simulink model "exp0303_sist_faltafaseterra"  (R2021b)
settings: Solver=ode23t  StartTime=0.0  StopTime=0.1  RelTol=1e-5  EnableMultiTasking=on
libraries: powerlib_extras x7, spsCurrentMeasurementLib x4, spsGroundLib x4, spsVoltageMeasurementLib x3, spsThreePhaseSeriesRLCBranchLib x2, spsThreePhaseSourceLib x1, spspowerguiLib x1
settings Model: Creator=alunos  LastModifiedBy=luang
settings SolverCC: AlgebraicLoopSolver=TrustRegion
settings DataIOCC: LimitDataPoints=on  SaveFormat=Array  SignalLoggingSaveFormat=ModelDataLogs  ReturnWorkspaceOutputs=off
settings OptimizationCC: ExpressionDepthLimit=2147483647  LifeSpan=inf
settings DebuggingCC: UnderspecifiedInitializationDetection=Classic  MergeDetectMultiDrivingBlocksExec=none  SolverPrmCheckMsg=warning  FcnCallInpInsideContextMsg=warning  StateNameClashWarn=warning  SFUnexpectedBacktrackingDiag=warning  SFNoUnconditionalDefaultTransitionDiag=warning  SFExecutionAtInitializationDiag=none  SFMachineParentedDataDiag=warning  ArithmeticOperatorsInVariantConditions=warning
settings HardwareCC: ProdBitPerPointer=32  ProdBitPerSizeT=32  ProdBitPerPtrDiffT=32  ProdLargestAtomicFloat=None  ProdIntDivRoundTo=Undefined  ProdEndianess=Unspecified  ProdWordSize=32  ProdHWDeviceType=32-bit Generic
settings ModelReferenceCC: PropagateSignalLabelsOutOfModel=off
settings SFSimCC: SimUseLocalCustomCode=off  CustomCodeUndefinedFunction=UseInterfaceOnly
settings RTWCC: RTWUseLocalCustomCode=off
settings CodeAppCC: StateflowObjectComments=on
settings GRTTargetCC: TargetLangStandard=C89/C90 (ANSI)  CombineOutputUpdateFcns=off  GRTInterface=on
settings ConfigComp: CovMetricSettings=dw  CovSaveCumulativeToWorkspaceVar=on  CovSaveSingleToWorkspaceVar=on  CovExternalEMLEnable=off

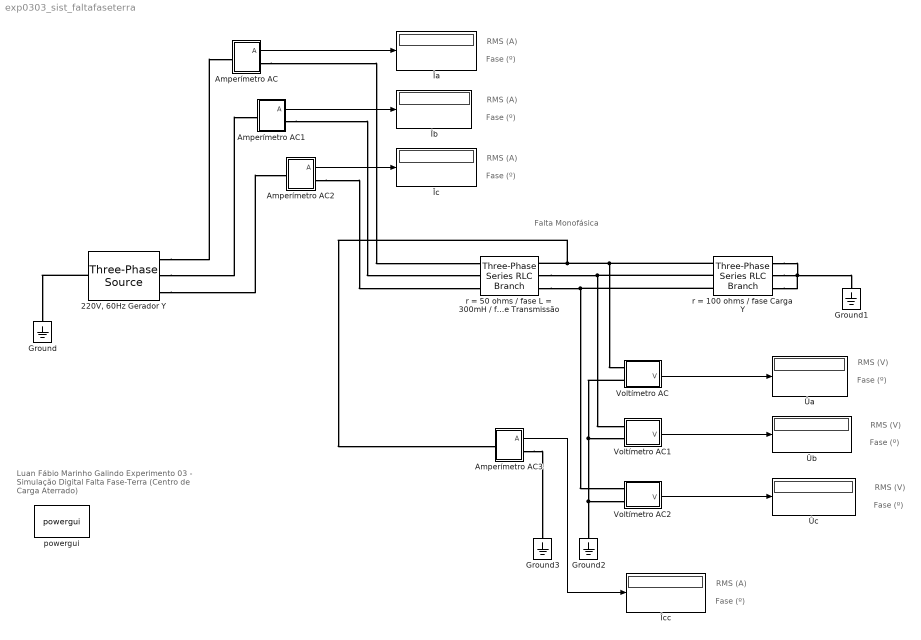
== system exp0303_sist_faltafaseterra ==
  note: Falta Monofásica
  note: RMS (A)
  note: Fase (º)
  note: RMS (A)
  note: Fase (º)
  note: RMS (A)
  note: Fase (º)
  note: RMS (V)
  note: Fase (º)
  note: RMS (V)
  note: Fase (º)
  note: RMS (V)
  note: Fase (º)
  note: Luan Fábio Marinho Galindo
      | Experimento 03 - Simulação Digital
      | Falta Fase-Terra (Centro de Carga Aterrado)
  note: RMS (A)
  note: Fase (º)
  "220V, 60Hz Gerador Y" : spsThreePhaseSourceLib/Three-Phase Source  InternalConnection=Yn  VoltagePhases=off  Voltage=220  PhaseAngle=90  Voltage_phases=[25e3 25e3 25e3]/sqrt(3)  PhaseAngles_phases=[0 -120 +120]  Frequency=60  NonIdealSource=on  SpecifyImpedance=off  Resistance=0.001  Inductance=0  ShortCircuitLevel=100e6  BaseVoltage=25e3  XRratio=7  BusType=swing  Pref=0  Qref=0  Prefabc=[10e3, 10e3, 10e3]  Qrefabc=[0, 0, 0]  Qmin=-inf  Qmax=inf
  Amperímetro AC : Subsystem
  Amperímetro AC1 : Subsystem
  Amperímetro AC2 : Subsystem
  Amperímetro AC3 : Subsystem
  Ground{,1..3} (4 alike) : spsGroundLib/Ground  LConnTagsString=a
  Voltímetro AC : Subsystem
  Voltímetro AC1 : Subsystem
  Voltímetro AC2 : Subsystem
  powergui : spspowerguiLib/powergui  Priority=1  SimulationMode=Continuous  SampleTime=50e-6  frequency=60  Iterations=50  frequencyindice=60  Pbase=100e6  ErrMax=1e-4  UnitsV=kV  UnitsW=MW  buscounter=0  FunctionMessages=off  echomessages=off  EnableUseOfTLC=off  CurrentSourceSwitches=on  DisableSnubberDevices=off  DisableRonSwitches=off  DisableVfSwitches=off  DisplayEquations=off  AutomaticDiscreteSolvers=off  SolverType=Tustin/Backward Euler (TBE)  Interpol=off  ExternalGateDelay=off  methode=off  Ts=100  x0status=blocks  SPID=off  SwTol=0  HookPort=off  NonlinearTolerance=1e-4  nMaxIteration=100  ContinueOnMaxIteration=off  RestoreLinks=warning  ResistiveCurrentMeasurement=off  Frange=[0:2:500]  Ylog=off  Xlog=on  ShowGrid=off  save=off  variable=ZData  structure=0  ZoomFFT=off  StartTime=0.0  cycles=1  DisplayStyle=1  fundamental=60  FreqAxis=off  MaxFrequency=1000  frequencyindicesteady=1  RmsSteady=1  display=off
  r = 100 ohms / fase Carga Y : spsThreePhaseSeriesRLCBranchLib/Three-Phase Series RLC Branch  LConnTagsString=A|B|C  RConnTagsString=A|B|C  BranchType=R  Resistance=100  Inductance=1e-3  Capacitance=1e-6  Measurements=None
  r = 50 ohms / fase L = 300mH / fase Linha de Transmissão : spsThreePhaseSeriesRLCBranchLib/Three-Phase Series RLC Branch  LConnTagsString=A|B|C  RConnTagsString=A|B|C  BranchType=RL  Resistance=50  Inductance=300e-3  Capacitance=1e-6  Measurements=None
  Îa : Display
      settings: Format=bank
  Îb : Display
      settings: Format=bank
  Îc : Display
      settings: Format=bank
  Îcc : Display
      settings: Format=bank
  Ûa : Display
      settings: Format=bank
  Ûb : Display
      settings: Format=bank
  Ûc : Display
      settings: Format=bank
  wires:
  Amperímetro AC/1(A) -> Îa/1
  Amperímetro AC1/1(A) -> Îb/1
  Amperímetro AC2/1(A) -> Îc/1
  Voltímetro AC/1(V) -> Ûa/1
  Voltímetro AC1/1(V) -> Ûb/1
  Voltímetro AC2/1(V) -> Ûc/1
  Amperímetro AC3/1(A) -> Îcc/1
  connections:
  "220V, 60Hz Gerador Y"/RConn1 -- Amperímetro AC/LConn1
  "220V, 60Hz Gerador Y"/RConn2 -- Amperímetro AC1/LConn1
  "220V, 60Hz Gerador Y"/RConn3 -- Amperímetro AC2/LConn1
  Amperímetro AC/RConn1 -- r = 50 ohms / fase L = 300mH / fase Linha de Transmissão/LConn1
  Amperímetro AC1/RConn1 -- r = 50 ohms / fase L = 300mH / fase Linha de Transmissão/LConn2
  Amperímetro AC2/RConn1 -- r = 50 ohms / fase L = 300mH / fase Linha de Transmissão/LConn3
  r = 100 ohms / fase Carga Y/RConn2 -- r = 100 ohms / fase Carga Y/RConn3 -- r = 100 ohms / fase Carga Y/RConn1 -- Ground1/LConn1
  Voltímetro AC/LConn1 -- r = 100 ohms / fase Carga Y/LConn1 -- r = 50 ohms / fase L = 300mH / fase Linha de Transmissão/RConn1 -- Amperímetro AC3/LConn1
  Voltímetro AC/LConn2 -- Voltímetro AC1/LConn2 -- Ground2/LConn1 -- Voltímetro AC2/LConn2
  "220V, 60Hz Gerador Y"/LConn1 -- Ground/LConn1
  r = 100 ohms / fase Carga Y/LConn3 -- r = 50 ohms / fase L = 300mH / fase Linha de Transmissão/RConn3 -- Voltímetro AC2/LConn1
  r = 50 ohms / fase L = 300mH / fase Linha de Transmissão/RConn2 -- Voltímetro AC1/LConn1 -- r = 100 ohms / fase Carga Y/LConn2
  Amperímetro AC3/RConn1 -- Ground3/LConn1

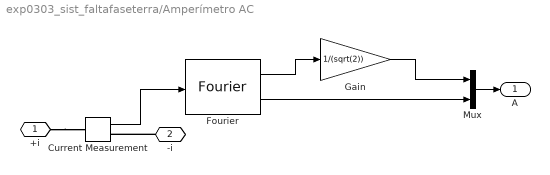
== system exp0303_sist_faltafaseterra/Amperímetro AC ==
  Current Measurement : spsCurrentMeasurementLib/Current Measurement  PhasorSimulation=off  OutputType=Complex  PSBequivalent=0
  Fourier : powerlib_extras/Measurements/Fourier  f1=60  n=1
      settings: SourceProductBaseCode=PS
  Gain : Gain  Gain=1/(sqrt(2))
  Mux : Mux  Inputs=2
  +i : PMIOPort  Side=Left
  -i : PMIOPort  Port=2  Side=Right
  A : Outport
  wires:
  Fourier/1 -> Gain/1
  Fourier/2 -> Mux/2
  Gain/1 -> Mux/1
  Current Measurement/1 -> Fourier/1
  Mux/1 -> A/1
  connections:
  +i/RConn1 -- Current Measurement/LConn1
  -i/RConn1 -- Current Measurement/RConn1

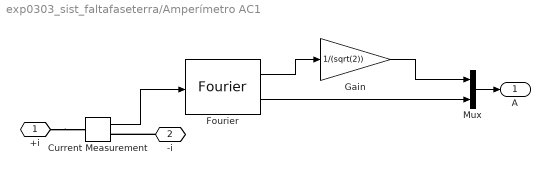
== system exp0303_sist_faltafaseterra/Amperímetro AC1 ==
  Current Measurement : spsCurrentMeasurementLib/Current Measurement  PhasorSimulation=off  OutputType=Complex  PSBequivalent=0
  Fourier : powerlib_extras/Measurements/Fourier  f1=60  n=1
      settings: SourceProductBaseCode=PS
  Gain : Gain  Gain=1/(sqrt(2))
  Mux : Mux  Inputs=2
  +i : PMIOPort  Side=Left
  -i : PMIOPort  Port=2  Side=Right
  A : Outport
  wires:
  Fourier/1 -> Gain/1
  Fourier/2 -> Mux/2
  Gain/1 -> Mux/1
  Current Measurement/1 -> Fourier/1
  Mux/1 -> A/1
  connections:
  +i/RConn1 -- Current Measurement/LConn1
  -i/RConn1 -- Current Measurement/RConn1

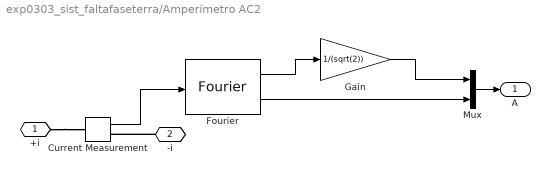
== system exp0303_sist_faltafaseterra/Amperímetro AC2 ==
  Current Measurement : spsCurrentMeasurementLib/Current Measurement  PhasorSimulation=off  OutputType=Complex  PSBequivalent=0
  Fourier : powerlib_extras/Measurements/Fourier  f1=60  n=1
      settings: SourceProductBaseCode=PS
  Gain : Gain  Gain=1/(sqrt(2))
  Mux : Mux  Inputs=2
  +i : PMIOPort  Side=Left
  -i : PMIOPort  Port=2  Side=Right
  A : Outport
  wires:
  Fourier/1 -> Gain/1
  Fourier/2 -> Mux/2
  Gain/1 -> Mux/1
  Current Measurement/1 -> Fourier/1
  Mux/1 -> A/1
  connections:
  +i/RConn1 -- Current Measurement/LConn1
  -i/RConn1 -- Current Measurement/RConn1

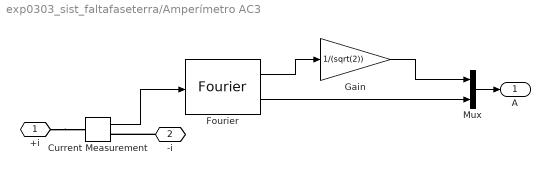
== system exp0303_sist_faltafaseterra/Amperímetro AC3 ==
  Current Measurement : spsCurrentMeasurementLib/Current Measurement  PhasorSimulation=off  OutputType=Complex  PSBequivalent=0
  Fourier : powerlib_extras/Measurements/Fourier  f1=60  n=1
      settings: SourceProductBaseCode=PS
  Gain : Gain  Gain=1/(sqrt(2))
  Mux : Mux  Inputs=2
  +i : PMIOPort  Side=Left
  -i : PMIOPort  Port=2  Side=Right
  A : Outport
  wires:
  Fourier/1 -> Gain/1
  Fourier/2 -> Mux/2
  Gain/1 -> Mux/1
  Current Measurement/1 -> Fourier/1
  Mux/1 -> A/1
  connections:
  +i/RConn1 -- Current Measurement/LConn1
  -i/RConn1 -- Current Measurement/RConn1

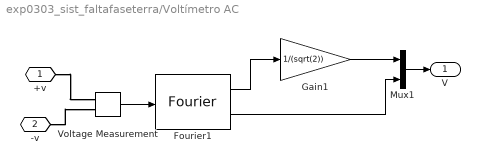
== system exp0303_sist_faltafaseterra/Voltímetro AC ==
  Fourier1 : powerlib_extras/Measurements/Fourier  f1=60  n=1
      settings: SourceProductBaseCode=PS
  Gain1 : Gain  Gain=1/(sqrt(2))
  Mux1 : Mux  Inputs=2
  Voltage Measurement : spsVoltageMeasurementLib/Voltage Measurement  PhasorSimulation=off  OutputType=Complex  PSBequivalent=0
  +v : PMIOPort  Side=Left
  -v : PMIOPort  Port=2  Side=Left
  V : Outport
  wires:
  Voltage Measurement/1 -> Fourier1/1
  Fourier1/1 -> Gain1/1
  Gain1/1 -> Mux1/1
  Fourier1/2 -> Mux1/2
  Mux1/1 -> V/1
  connections:
  +v/RConn1 -- Voltage Measurement/LConn1
  -v/RConn1 -- Voltage Measurement/LConn2

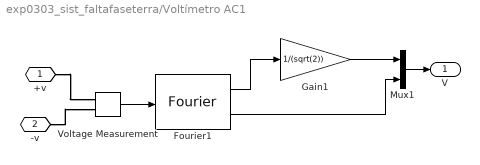
== system exp0303_sist_faltafaseterra/Voltímetro AC1 ==
  Fourier1 : powerlib_extras/Measurements/Fourier  f1=60  n=1
      settings: SourceProductBaseCode=PS
  Gain1 : Gain  Gain=1/(sqrt(2))
  Mux1 : Mux  Inputs=2
  Voltage Measurement : spsVoltageMeasurementLib/Voltage Measurement  PhasorSimulation=off  OutputType=Complex  PSBequivalent=0
  +v : PMIOPort  Side=Left
  -v : PMIOPort  Port=2  Side=Left
  V : Outport
  wires:
  Voltage Measurement/1 -> Fourier1/1
  Fourier1/1 -> Gain1/1
  Gain1/1 -> Mux1/1
  Fourier1/2 -> Mux1/2
  Mux1/1 -> V/1
  connections:
  +v/RConn1 -- Voltage Measurement/LConn1
  -v/RConn1 -- Voltage Measurement/LConn2

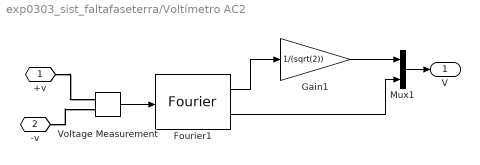
== system exp0303_sist_faltafaseterra/Voltímetro AC2 ==
  Fourier1 : powerlib_extras/Measurements/Fourier  f1=60  n=1
      settings: SourceProductBaseCode=PS
  Gain1 : Gain  Gain=1/(sqrt(2))
  Mux1 : Mux  Inputs=2
  Voltage Measurement : spsVoltageMeasurementLib/Voltage Measurement  PhasorSimulation=off  OutputType=Complex  PSBequivalent=0
  +v : PMIOPort  Side=Left
  -v : PMIOPort  Port=2  Side=Left
  V : Outport
  wires:
  Voltage Measurement/1 -> Fourier1/1
  Fourier1/1 -> Gain1/1
  Gain1/1 -> Mux1/1
  Fourier1/2 -> Mux1/2
  Mux1/1 -> V/1
  connections:
  +v/RConn1 -- Voltage Measurement/LConn1
  -v/RConn1 -- Voltage Measurement/LConn2
